simulink model "Kalman_Filterr"  (R2022b)
settings: Solver=ode1  StartTime=0.0  StopTime=inf  FixedStep=0.002  RelTol=1e-3  EnableMultiTasking=on
values from neighbouring files (symbols this model uses):
  A = [0 0 1 0 ... (first row only)    [LQR.m]
  B = [0; 0; Km*J2_star/(Rm*Jt); Km*c/(Rm*Jt)]    [LQR.m]
  C = [1 0 0 0 ... (first row only)    [LQR.m]
  D = [0;0]    [LQR.m]
  Kalfa = 0.2    [LQR.m]
  Ktheta = 0.5    [LQR.m]
  Kw = 2    [LQR.m]
  Q = 1    [LQR.m]
  R = 0.1    [LQR.m]
  Ts = 0.002    [LQR.m]
undefined symbols (not defined in the file or in its folder): Continuous, HIL, K, qc_get_step_size, Time
libraries: simulink_extras x3, simulink x3, quarc_library x3, sharedTrackingLibrary x1, ctrlSharedLib x1
settings Model: SimulationMode=external  ExtModeTrigDuration=5000  Creator=MLevis  LastModifiedBy=Utente
settings SolverCC: AlgebraicLoopSolver=TrustRegion  PositivePriorityOrder=on
settings DataIOCC: LimitDataPoints=on  SaveFormat=Array  SignalLoggingSaveFormat=ModelDataLogs  ReturnWorkspaceOutputs=off
settings OptimizationCC: BooleanDataType=off  OptimizeBlockIOStorage=off  BufferReuse=off  GlobalBufferReuse=off  ExpressionFolding=off  ExpressionDepthLimit=2147483647  LocalBlockOutputs=off  InitFltsAndDblsToZero=on  OptimizeDataStoreBuffers=off  BusAssignmentInplaceUpdate=off
settings DebuggingCC: SaveWithParameterizedLinksMsg=none  UnderspecifiedInitializationDetection=Classic  MergeDetectMultiDrivingBlocksExec=none  SignalResolutionControl=TryResolveAllWithWarning  MultiTaskDSMMsg=warning  MultiTaskCondExecSysMsg=none  FcnCallInpInsideContextMsg=warning  UnconnectedInputMsg=warning  UnconnectedOutputMsg=warning  UnconnectedLineMsg=warning  StateNameClashWarn=warning  SFUnexpectedBacktrackingDiag=warning  SFNoUnconditionalDefaultTransitionDiag=warning  SFExecutionAtInitializationDiag=none  SFMachineParentedDataDiag=warning  ArithmeticOperatorsInVariantConditions=warning
settings HardwareCC: TargetHWDeviceType=32-bit Generic
settings ModelReferenceCC: EnableRefExpFcnMdlSchedulingChecks=on  PropagateSignalLabelsOutOfModel=off
settings SFSimCC: SimUseLocalCustomCode=off  SimParseCustomCode=off  CustomCodeUndefinedFunction=UseInterfaceOnly
settings RTWCC: Description=QUARC Win64 Target Using Toolchain  SystemTargetFile=quarc_win64.tlc  TemplateMakefile=quarc_default_tmf  RTWUseLocalCustomCode=off  Toolchain=QUARC win64 | nmake (64-bit Windows)  BuildConfiguration=Faster Runs
settings CodeAppCC: StateflowObjectComments=on
settings STFCustomTargetCC: ConcurrentExecutionCompliant=on  GRTInterface=on  UseToolchainInfoCompliant=on  SystemTargetFile=quarc_win64.tlc
settings GRTTargetCC: TargetLangStandard=C89/C90 (ANSI)  ParMdlRefBuildCompliant=off  CompOptLevelCompliant=off  CombineOutputUpdateFcns=off  MatFileLogging=off  CPPClassGenCompliant=off  GRTInterface=on  ExtMode=on  ExtModeMexFile=quarc_comm
settings ConfigComp: CovMetricSettings=dw  CovSaveCumulativeToWorkspaceVar=on  CovSaveSingleToWorkspaceVar=on  CovExternalEMLEnable=off  CovSFcnEnable=off

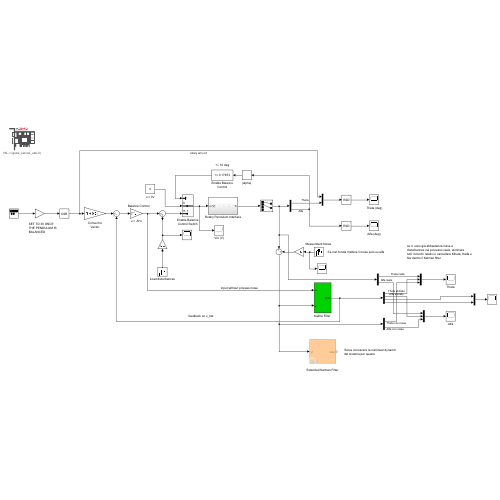
[thumbnail: Simulink's stored preview of the top-level diagram]
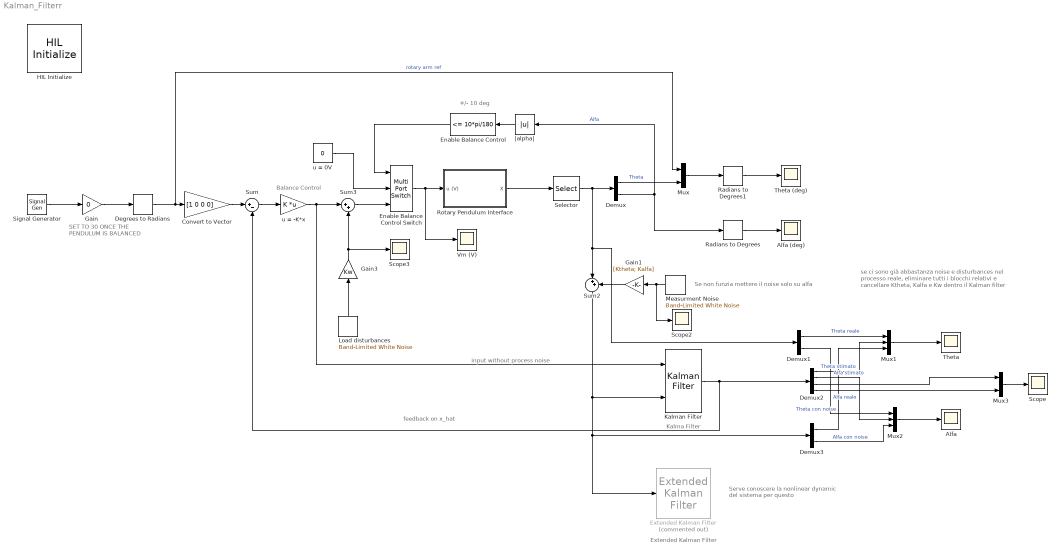
== system Kalman_Filterr ==
  note: feedback on x_hat
  note: Serve conoscere la nonlinear dynamic
      | del sistema per questo
  note: Extended Kalman Filter
  note: se ci sono già abbastanza noise e
      | disturbances nel processo reale, eliminare
      | tutti i blocchi relativi e cancellare Ktheta, Kalfa e
      | Kw dentro il Kalman filter
  note: input without process noise
  note: Kalma Filter
  note: Se non funzia mettere il noise solo su alfa
  note: SET TO 30 ONCE
      | THE PENDULUM IS
      | BALANCED
  note: +/- 10 deg
  note: Balance Control
  " Theta (deg)" : Scope
  Alfa : Scope
  Alfa (deg) : Scope
  Convert to Vector : Gain  Gain=[1 0 0 0]
  Degrees to Radians : simulink_extras/Transformations/Degrees to Radians
  Demux : Demux  Outputs=2
  Demux1 : Demux  Outputs=2
  Demux2 : Demux
  Demux3 : Demux  Outputs=2
  Enable Balance Control : simulink/Logic and Bit Operations/Compare To Constant  relop=<=  const=10*pi/180  OutDataTypeStr=uint8  ZeroCross=off
  Enable Balance Control Switch : MultiPortSwitch  DataPortOrder=Zero-based contiguous  Inputs=2  zeroidx=on  SaturateOnIntegerOverflow=off  InputSameDT=off
  Extended Kalman Filter : sharedTrackingLibrary/Extended Kalman Filter  Commented=on  StateTransitionFcn=myStateTransitionFcn  HasStateTransitionJacobianFcn=off  HasAdditiveProcessNoise=Additive  ProcessNoise=diag([Kw^2*Q 0 0 0])  HasTimeVaryingProcessNoise=off  HasStateTransitionFcnExtraArgument=0  InitialState=[0; 0]  InitialStateCovariance=1e-3  MeasurementFcn1=myMeasurementFcn  HasMeasurementJacobianFcn1=off  HasMeasurementEnablePort1=off  HasAdditiveMeasurementNoise1=Additive  MeasurementNoise1=diag([Ktheta^2*R Kalfa^2*R])  HasTimeVaryingMeasurementNoise1=off  HasMeasurementFcnExtraArgument1=0  HasMeasurementWrapping1=off  MeasurementFcn2=myMeasurementFcn  HasMeasurementJacobianFcn2=off  HasMeasurementEnablePort2=off  HasAdditiveMeasurementNoise2=Additive  MeasurementNoise2=1  HasTimeVaryingMeasurementNoise2=off  HasMeasurementFcnExtraArgument2=0  HasMeasurementWrapping2=off  MeasurementFcn3=myMeasurementFcn  HasMeasurementJacobianFcn3=off  HasMeasurementEnablePort3=off  HasAdditiveMeasurementNoise3=Additive  MeasurementNoise3=1  HasTimeVaryingMeasurementNoise3=off  HasMeasurementFcnExtraArgument3=0  HasMeasurementWrapping3=off  MeasurementFcn4=myMeasurementFcn  HasMeasurementJacobianFcn4=off  HasMeasurementEnablePort4=off  HasAdditiveMeasurementNoise4=Additive  MeasurementNoise4=1  HasTimeVaryingMeasurementNoise4=off  HasMeasurementFcnExtraArgument4=0  HasMeasurementWrapping4=off  MeasurementFcn5=myMeasurementFcn  HasMeasurementJacobianFcn5=off  HasMeasurementEnablePort5=off  HasAdditiveMeasurementNoise5=Additive  MeasurementNoise5=1  HasTimeVaryingMeasurementNoise5=off  HasMeasurementFcnExtraArgument5=0  HasMeasurementWrapping5=off  EnableMultirate=off  StateTransitionFcnSampleTime=1  MeasurementFcn1SampleTime=1  MeasurementFcn2SampleTime=1  MeasurementFcn3SampleTime=1  MeasurementFcn4SampleTime=1  MeasurementFcn5SampleTime=1  UseCurrentEstimator=on  OutputStateCovariance=off  DataType=double  SampleTime=1  NumberOfMeasurements=1
  Gain : Gain  Gain=0
  Gain1 : Gain  Gain=[Ktheta; Kalfa]
  Gain3 : Gain  Gain=Kw
  HIL Initialize : quarc_library/Data Acquisition/Generic/Configuration/HIL Initialize  object_name=HIL-1  board_type=qube_servo2_usb  board_number=0  board_options=""  exclusive=off  active=off  hardware_clocks=[0]  clock_modes=[]  initial_clock_frequencies=[]  set_clock_params_at_start=off  set_clock_params_at_switch_in=off  set_clock_frequencies_at_start=off  set_clock_frequencies_at_switch_in=off  analog_input_channels=[0]  analog_input_configurations=[]  analog_input_maximums=3  analog_input_minimums=-3  set_analog_input_params_at_start=off  set_analog_input_params_at_switch_in=off  analog_output_channels=[0]  analog_output_maximums=15  analog_output_minimums=-15  initial_analog_outputs=[0]  final_analog_outputs=[0]  watchdog_analog_outputs=0  set_analog_output_params_at_start=off  set_analog_output_params_at_switch_in=off  set_analog_outputs_at_start=on  set_analog_outputs_at_switch_in=off  set_analog_outputs_at_terminate=on  set_analog_outputs_at_switch_out=off  set_analog_outputs_on_watchdog=on  digital_input_channels=[]  digital_output_channels=[0]  digital_output_configuration=[]  initial_digital_outputs=[1]  final_digital_outputs=[0]  watchdog_digital_outputs=[0]  set_digital_output_params_at_start=off  set_digital_output_params_at_switch_in=off  set_digital_outputs_at_start=on  set_digital_outputs_at_switch_in=off  set_digital_outputs_at_terminate=on  set_digital_outputs_at_switch_out=off  set_digital_outputs_on_watchdog=on  encoder_channels=[0:1]  quadrature=[4]  encoder_filter_frequency=[]  initial_encoder_counts=[0]  set_encoder_params_at_start=off  set_encoder_params_at_switch_in=off  set_encoder_counts_at_start=on  set_encoder_counts_at_switch_in=off  pwm_channels=[]  pwm_modes=[]  pwm_frequency=[]  pwm_configuration=[]  pwm_alignment=[]  pwm_polarity=[]  pwm_leading_deadband=[]  pwm_trailing_deadband=[]  initial_pwm_outputs=[]  final_pwm_outputs=[]  watchdog_pwm_outputs=[]  set_pwm_params_at_start=off  set_pwm_params_at_switch_in=off  set_pwm_outputs_at_start=off  set_pwm_outputs_at_switch_in=off  set_pwm_outputs_at_terminate=off  set_pwm_outputs_at_switch_out=off  set_pwm_outputs_on_watchdog=off  other_output_channels=[11000:11002]  initial_other_outputs=[0 1 0]  final_other_outputs=[1 0 0]  watchdog_other_outputs=[0 0 1]  set_other_outputs_at_start=on  set_other_outputs_at_switch_in=off  set_other_outputs_at_terminate=on  set_other_outputs_at_switch_out=off  set_other_outputs_on_watchdog=on
  Kalman Filter : ctrlSharedLib/Kalman Filter  TimeDomain=Continuous-Time  UseCurrentEstimator=on  ModelSource=Individual A, B, C, D matrices  ModelSourceVariable=ss(0.95,1,1,0,1)  A=A  B=B  C=C  D=D  NumberOfStates=1  NumberOfInputs=1  NumberOfOutputs=1  InitialEstimateSource=Dialog  X0=[0;0;0;0]  P0=10  UseK=off  UseGH=off  NumberOfProcessNoiseInputs=1  G=1  TimeInvariantG=on  H=0  TimeInvariantH=on  Q=diag([Kw^2*Q 0 0 0])  TimeInvariantQ=on  R=diag([Ktheta^2*R Kalfa^2*R])  TimeInvariantR=on  N=0  TimeInvariantN=on  AddInputPort=on  AddEnablePort=off  OutputEstimatedY=off  OutputP=off  Ts=-1
  Load disturbances : simulink/Sources/Band-Limited White Noise  Cov=Q*Ts  Ts=0.02  seed=[23341]
  "Measurment Noise " : simulink/Sources/Band-Limited White Noise  Cov=R*Ts  Ts=Ts  seed=[12537]
  Mux : Mux  Inputs=2
  Mux1 : Mux  Inputs=3
  Mux2 : Mux  Inputs=3
  Mux3 : Mux  Inputs=2
  Radians to Degrees : simulink_extras/Transformations/Radians to Degrees
  Radians to Degrees1 : simulink_extras/Transformations/Radians to Degrees
  Rotary Pendulum Interface : Subsystem
  Scope : Scope
  Scope2 : Scope
  Scope3 : Scope
  Selector : Selector  InputPortWidth=4  IndexOptions=Index vector (dialog)  Indices=[1 2]  OutputSizes=1
  Signal Generator : SignalGenerator  WaveForm=square  Frequency=0.125
  Sum : Sum  Inputs=|+-
  Sum2 : Sum  Inputs=|++
  Sum3 : Sum  Inputs=|++
  Theta : Scope
  Vm (V) : Scope
  u = -K*x : Gain  Gain=K  Multiplication=Matrix(K*u)
  u = 0V : Constant  Value=0
  |alpha| : Abs  SaturateOnIntegerOverflow=off
  wires:
  |alpha|/1 -> Enable Balance Control/1
  Enable Balance Control/1 -> Enable Balance Control Switch/1
  Sum/1 -> u = -K*x/1
  Convert to Vector/1 -> Sum/1
  Radians to Degrees/1 -> Alfa (deg)/1
  Radians to Degrees1/1 -> " Theta (deg)"/1
  Enable Balance Control Switch/1 -> Vm (V)/1, Rotary Pendulum Interface/1(u (V))
  u = 0V/1 -> Enable Balance Control Switch/2
  Signal Generator/1 -> Gain/1
  Gain/1 -> Degrees to Radians/1
  Degrees to Radians/1 -> Mux/1, Convert to Vector/1  "rotary arm ref"
  Mux/1 -> Radians to Degrees1/1
  Rotary Pendulum Interface/1(X) -> Selector/1
  Selector/1 -> Demux/1, Demux1/1, Sum2/1
  Demux/1 -> Mux/2  "Theta"
  Demux/2 -> Radians to Degrees/1, |alpha|/1  "Alfa"
  u = -K*x/1 -> Kalman Filter/1, Sum3/1
  "Measurment Noise "/1 -> Scope2/1, Gain1/1
  Gain1/1 -> Sum2/2
  Sum2/1 -> Extended Kalman Filter/1, Demux3/1, Kalman Filter/2
  Gain3/1 -> Scope3/1, Sum3/2
  Load disturbances/1 -> Gain3/1
  Sum3/1 -> Enable Balance Control Switch/3
  Kalman Filter/1 -> Sum/2, Demux2/1
  Demux1/1 -> Mux1/1  "Theta reale"
  Demux2/1 -> Mux1/2  "Theta stimato"
  Demux3/1 -> Mux1/3  "Theta con noise"
  Mux1/1 -> Theta/1
  Demux1/2 -> Mux2/1  "Alfa reale"
  Demux2/2 -> Mux2/2  "Alfa stimato"
  Demux3/2 -> Mux2/3  "Alfa con noise"
  Mux2/1 -> Alfa/1
  Demux2/3 -> Mux3/1
  Demux2/4 -> Mux3/2
  Mux3/1 -> Scope/1

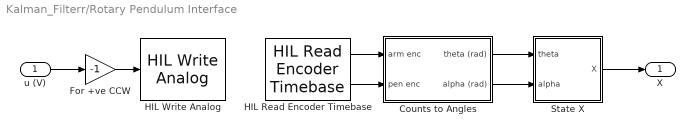
== system Kalman_Filterr/Rotary Pendulum Interface ==
  u (V) : Inport
  Counts to Angles : Subsystem
  For +ve CCW : Gain  Gain=-1
  HIL Read Encoder Timebase : quarc_library/Data Acquisition/Generic/Timebases/HIL Read Encoder Timebase  object_name=HIL-1  clock=0  channels=[0:1]  active=on  vector_output=off  data_type_mode=Inherit via back propagation  data_type=double  overflow_mode=Error on overflow  samples_in_buffer=max(ceil(1/qc_get_step_size), 1)
  HIL Write Analog : quarc_library/Data Acquisition/Generic/Immediate I//O/HIL Write Analog  object_name=HIL-1  channels=0  sample_time=-1  active=off  vector_input=off
  State X : Subsystem
  X : Outport  VectorParamsAs1DForOutWhenUnconnected=off
  wires:
  u (V)/1 -> For +ve CCW/1
  HIL Read Encoder Timebase/2 -> Counts to Angles/2(pen enc)
  For +ve CCW/1 -> HIL Write Analog/1
  HIL Read Encoder Timebase/1 -> Counts to Angles/1(arm enc)
  Counts to Angles/2(alpha (rad)) -> State X/2(alpha)
  Counts to Angles/1(theta (rad)) -> State X/1(theta)
  State X/1(X) -> X/1

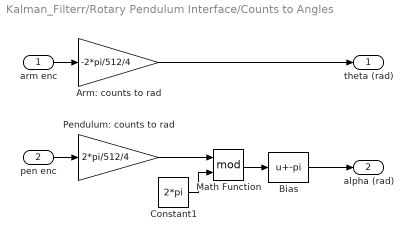
== system Kalman_Filterr/Rotary Pendulum Interface/Counts to Angles ==
  arm enc : Inport
  pen enc : Inport  Port=2
  Arm: counts to rad : Gain  Gain=-2*pi/512/4
  Bias : Bias  Bias=-pi  SaturateOnIntegerOverflow=off
  Constant1 : Constant  Value=2*pi
  Math Function : Math  Operator=mod  SignedPower=on
  Pendulum: counts to rad : Gain  Gain=2*pi/512/4
  theta (rad) : Outport  VectorParamsAs1DForOutWhenUnconnected=off
  alpha (rad) : Outport  Port=2  VectorParamsAs1DForOutWhenUnconnected=off
  wires:
  pen enc/1 -> Pendulum: counts to rad/1
  arm enc/1 -> Arm: counts to rad/1
  Math Function/1 -> Bias/1
  Constant1/1 -> Math Function/2
  Pendulum: counts to rad/1 -> Math Function/1
  Arm: counts to rad/1 -> theta (rad)/1
  Bias/1 -> alpha (rad)/1

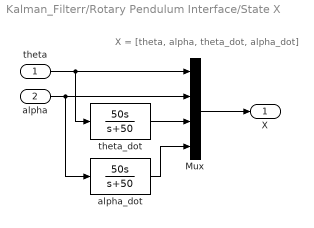
== system Kalman_Filterr/Rotary Pendulum Interface/State X ==
  note: X = [theta, alpha, theta_dot, alpha_dot]
  theta : Inport
  alpha : Inport  Port=2
  Mux : Mux
  alpha_dot : TransferFcn  Numerator=[50 0]  Denominator=[1 50]
  theta_dot : TransferFcn  Numerator=[50 0]  Denominator=[1 50]
  X : Outport  VectorParamsAs1DForOutWhenUnconnected=off
  wires:
  theta_dot/1 -> Mux/3
  alpha_dot/1 -> Mux/4
  alpha/1 -> Mux/2, alpha_dot/1
  Mux/1 -> X/1
  theta/1 -> Mux/1, theta_dot/1
